simulink model "gleit_komma3"  (Simulink 7.8)
settings: Solver=ode45  StartTime=0.0  StopTime=10.0  RelTol=1e-3
settings Model: Creator=svenhoffmann  LastModifiedBy=josef  ExtModeAutoUpdateStatusClock=off
settings DataIOCC: SignalLoggingName=sigsOut
settings OptimizationCC: InlineInvariantSignals=on  InitFltsAndDblsToZero=on
settings DebuggingCC: SaveWithParameterizedLinksMsg=none  SignalResolutionControl=TryResolveAllWithWarning  SolverPrmCheckMsg=none  MultiTaskDSMMsg=warning  MultiTaskCondExecSysMsg=none  FcnCallInpInsideContextMsg=Use local settings  StrictBusMsg=None
settings HardwareCC: TargetUnknown=on
settings RTWCC: IncludeERTFirstTime=on
settings GRTTargetCC: TargetFcnLib=ansi_tfl_tmw.mat

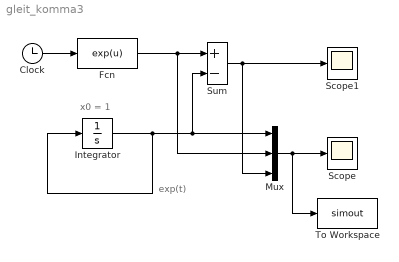
== system gleit_komma3 ==
  note: x0 = 1
  note: exp(t)
  Clock : Clock
  Fcn : Fcn  Expr=exp(u)
  Integrator : Integrator  InitialCondition=1
  Mux : Mux  Inputs=3
  Scope : Scope
  Scope1 : Scope
  Sum : Sum  Inputs=+-  SaturateOnIntegerOverflow=on
  To Workspace : ToWorkspace  VariableName=simout  SampleTime=-1  SaveFormat=Structure With Time
  wires:
  Integrator/1 -> Sum/2, Mux/1, Integrator/1
  Clock/1 -> Fcn/1
  Fcn/1 -> Sum/1, Mux/2
  Sum/1 -> Scope1/1, Mux/3
  Mux/1 -> Scope/1, To Workspace/1
